simulink subsystem "Batteri"  (R2020b)
settings: Solver=VariableStepAuto  StartTime=0.0  StopTime=10.0  RelTol=1e-3
libraries: fl_lib x76, ee_lib x27, nesl_utility x2
(part 1 of 2)
settings Model: Creator=David  LastModifiedBy=Sixten

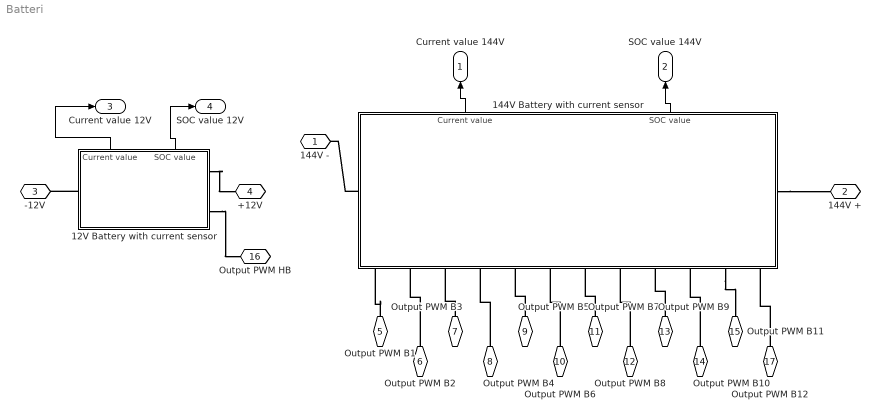
== system Batteri ==
  " 144V Battery with current sensor" : Subsystem
      settings: PortSchema="{\"entries\":[{\"content\":{\"sides\":[{\"content\":{\"connectorIds\":[\"LConn1\"]},\"type\":\"ConnectorPlacement.EquallySpacedRectSide\",\"uuid\":\"de94b407-ac45-4158-bf87-f7f71205b953\"},{\"content\":{\"connectorIds\":[\"RConn1\"],\"side\":\"RIGHT\"},\"type\":\"ConnectorPlacement.EquallySpacedRectSide\",\"uuid\":\"5f37bfd3-1f83-41a2-8e4c-c028e2b46b1f\"},{\"content\":{\"connectorIds\":[\"Out1\",\"Out2\"],\"side\":\"TOP\"},\"type\":\"ConnectorPlacement.EquallySpacedRectSide\",\"uuid\":\"a2342012-b85c-4526-9142-351f25c37e79\"},{\"content\":{\"connectorIds\":[\"RConn2\",\"RConn3\",\"RConn4\",\"RConn5\",\"RConn6\",\"RConn7\",\"RConn8\",\"RConn9\",\"RConn10\",\"RConn11\",\"RConn12\",\"RConn13\"],\"side\":\"BOTTOM\"},\"type\":\"ConnectorPlacement.EquallySpacedRectSide\",\"uuid\":\"61a274a5-577d-4bb8-8dc8-b17a7a1decde\"},{\"content\":{\"connectorIds\":[],\"side\":\"HIDDEN\"},\"type\":\"ConnectorPlacement.EquallySpacedRectSide\",\"uuid\":\"c9b59ba9-0057-4e9f-a00a-12995deaa940\"}]},\"type\":\"ConnectorPlacement.EquallySpacedConnector\",\"uuid\":\"0aadbf9b-8ffe-4e11-88ee-655997b921c3\"}],\"packageUris\":[\"http://schema.mathworks.com/mf0/Connector/R2020b\"],\"version\":\"1.0\"}"
  12V Battery with current sensor : Subsystem
      settings: PortSchema="{\"entries\":[{\"content\":{\"sides\":[{\"content\":{\"connectorIds\":[\"LConn1\"]},\"type\":\"ConnectorPlacement.EquallySpacedRectSide\",\"uuid\":\"de94b407-ac45-4158-bf87-f7f71205b953\"},{\"content\":{\"connectorIds\":[\"RConn1\",\"RConn2\"],\"side\":\"RIGHT\"},\"type\":\"ConnectorPlacement.EquallySpacedRectSide\",\"uuid\":\"5f37bfd3-1f83-41a2-8e4c-c028e2b46b1f\"},{\"content\":{\"connectorIds\":[\"Out1\",\"Out2\"],\"side\":\"TOP\"},\"type\":\"ConnectorPlacement.EquallySpacedRectSide\",\"uuid\":\"a2342012-b85c-4526-9142-351f25c37e79\"},{\"content\":{\"connectorIds\":[],\"side\":\"BOTTOM\"},\"type\":\"ConnectorPlacement.EquallySpacedRectSide\",\"uuid\":\"fa1d5bca-3a30-4491-90b2-05abb2f1cee1\"},{\"content\":{\"connectorIds\":[],\"side\":\"HIDDEN\"},\"type\":\"ConnectorPlacement.EquallySpacedRectSide\",\"uuid\":\"c9b59ba9-0057-4e9f-a00a-12995deaa940\"}]},\"type\":\"ConnectorPlacement.EquallySpacedConnector\",\"uuid\":\"0aadbf9b-8ffe-4e11-88ee-655997b921c3\"}],\"packageUris\":[\"http://schema.mathworks.com/mf0/Connector/R2020b\"],\"version\":\"1.0\"}"
  144V - : PMIOPort  Side=Left
  144V + : PMIOPort  Port=2  Side=Right
  -12V : PMIOPort  Port=3  Side=Left
  +12V : PMIOPort  Port=4  Side=Right
  Output PWM B1 : PMIOPort  Port=5  Side=Right
  Output PWM B2 : PMIOPort  Port=6  Side=Right
  Output PWM B3 : PMIOPort  Port=7  Side=Right
  Output PWM B4 : PMIOPort  Port=8  Side=Right
  Output PWM B5 : PMIOPort  Port=9  Side=Right
  Output PWM B6 : PMIOPort  Port=10  Side=Right
  Output PWM B7 : PMIOPort  Port=11  Side=Right
  Output PWM B8 : PMIOPort  Port=12  Side=Right
  Output PWM B9 : PMIOPort  Port=13  Side=Right
  Output PWM B10 : PMIOPort  Port=14  Side=Right
  Output PWM B11 : PMIOPort  Port=15  Side=Right
  Output PWM HB : PMIOPort  Port=16  Side=Right
  Output PWM B12 : PMIOPort  Port=17  Side=Right
  Current value 144V : Outport
  SOC value 144V : Outport  Port=2
  Current value 12V : Outport  Port=3
  SOC value 12V : Outport  Port=4
  wires:
  " 144V Battery with current sensor"/1(Current value) -> Current value 144V/1
  12V Battery with current sensor/1(Current value) -> Current value 12V/1
  12V Battery with current sensor/2(SOC value) -> SOC value 12V/1
  " 144V Battery with current sensor"/2(SOC value) -> SOC value 144V/1
  connections:
  " 144V Battery with current sensor"/RConn1 -- 144V +/RConn1
  " 144V Battery with current sensor"/LConn1 -- 144V -/RConn1
  12V Battery with current sensor/LConn1 -- -12V/RConn1
  12V Battery with current sensor/RConn1 -- +12V/RConn1
  Output PWM B1/RConn1 -- " 144V Battery with current sensor"/RConn2
  Output PWM B2/RConn1 -- " 144V Battery with current sensor"/RConn3
  Output PWM B3/RConn1 -- " 144V Battery with current sensor"/RConn4
  Output PWM B4/RConn1 -- " 144V Battery with current sensor"/RConn5
  Output PWM B5/RConn1 -- " 144V Battery with current sensor"/RConn6
  Output PWM B6/RConn1 -- " 144V Battery with current sensor"/RConn7
  Output PWM B7/RConn1 -- " 144V Battery with current sensor"/RConn8
  Output PWM B8/RConn1 -- " 144V Battery with current sensor"/RConn9
  Output PWM B9/RConn1 -- " 144V Battery with current sensor"/RConn10
  Output PWM B10/RConn1 -- " 144V Battery with current sensor"/RConn11
  " 144V Battery with current sensor"/RConn12 -- Output PWM B11/RConn1
  12V Battery with current sensor/RConn2 -- Output PWM HB/RConn1
  Output PWM B12/RConn1 -- " 144V Battery with current sensor"/RConn13

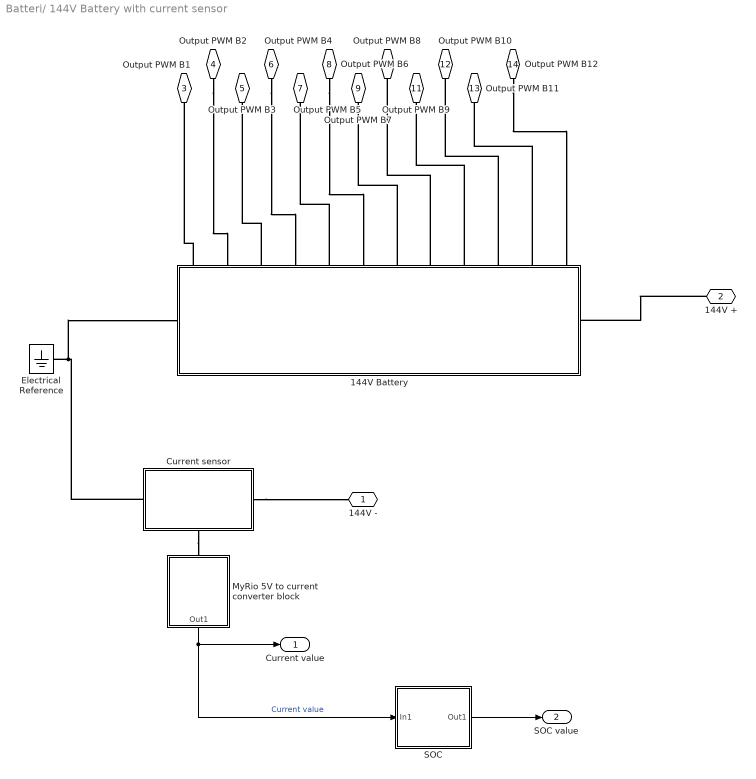
== system Batteri/ 144V Battery with current sensor ==
  " SOC" : Subsystem
  144V Battery : Subsystem
      settings: PortSchema="{\"entries\":[{\"content\":{\"sides\":[{\"content\":{\"connectorIds\":[\"LConn1\"]},\"type\":\"ConnectorPlacement.EquallySpacedRectSide\",\"uuid\":\"e99ced6f-69e8-4252-8471-6cdb96ceb2b2\"},{\"content\":{\"connectorIds\":[\"RConn1\"],\"side\":\"RIGHT\"},\"type\":\"ConnectorPlacement.EquallySpacedRectSide\",\"uuid\":\"43ce9788-4860-4398-aee6-6e594bef3b24\"},{\"content\":{\"connectorIds\":[\"LConn2\",\"LConn3\",\"LConn4\",\"LConn5\",\"LConn6\",\"LConn7\",\"LConn8\",\"LConn9\",\"LConn10\",\"LConn11\",\"LConn12\",\"LConn13\"],\"side\":\"TOP\"},\"type\":\"ConnectorPlacement.EquallySpacedRectSide\",\"uuid\":\"c38ed088-7784-4d04-84fd-2543a273ac23\"},{\"content\":{\"connectorIds\":[],\"side\":\"HIDDEN\"},\"type\":\"ConnectorPlacement.EquallySpacedRectSide\",\"uuid\":\"e037fcb5-e400-4ff2-9ee1-c6dab5a4f657\"}]},\"type\":\"ConnectorPlacement.EquallySpacedConnector\",\"uuid\":\"0126c910-ab8b-459c-9426-4e860af266e9\"}],\"packageUris\":[\"http://schema.mathworks.com/mf0/Connector/R2020b\"],\"version\":\"1.0\"}"
  Current sensor : Subsystem
      settings: PortSchema="{\"entries\":[{\"content\":{\"sides\":[{\"content\":{\"connectorIds\":[\"LConn1\"]},\"type\":\"ConnectorPlacement.EquallySpacedRectSide\",\"uuid\":\"83570808-fc29-4e6a-be28-aa8d0eabb79f\"},{\"content\":{\"connectorIds\":[\"RConn1\"],\"side\":\"RIGHT\"},\"type\":\"ConnectorPlacement.EquallySpacedRectSide\",\"uuid\":\"416c4cd8-a069-48b3-a3c7-74116419a4db\"},{\"content\":{\"connectorIds\":[],\"side\":\"TOP\"},\"type\":\"ConnectorPlacement.EquallySpacedRectSide\",\"uuid\":\"a4fb3738-5515-4a74-8adf-a2dd979befdd\"},{\"content\":{\"connectorIds\":[\"RConn2\"],\"side\":\"BOTTOM\"},\"type\":\"ConnectorPlacement.EquallySpacedRectSide\",\"uuid\":\"ad628acf-3503-4419-88b3-b3eb14bb30ce\"},{\"content\":{\"connectorIds\":[],\"side\":\"HIDDEN\"},\"type\":\"ConnectorPlacement.EquallySpacedRectSide\",\"uuid\":\"b744c287-8e60-4db7-938e-bc5b63a55d48\"}]},\"type\":\"ConnectorPlacement.EquallySpacedConnector\",\"uuid\":\"a4a86a7b-faa9-4dcc-948f-f4075230c4ff\"}],\"packageUris\":[\"http://schema.mathworks.com/mf0/Connector/R2020b\"],\"version\":\"1.0\"}"
  Electrical Reference : fl_lib/Electrical/Electrical Elements/Electrical Reference
  MyRio 5V to current converter block : Subsystem
  144V - : PMIOPort  Side=Left
  144V + : PMIOPort  Port=2  Side=Right
  Output PWM B1 : PMIOPort  Port=3  Side=Right
  Output PWM B2 : PMIOPort  Port=4  Side=Right
  Output PWM B3 : PMIOPort  Port=5  Side=Right
  Output PWM B4 : PMIOPort  Port=6  Side=Right
  Output PWM B5 : PMIOPort  Port=7  Side=Right
  Output PWM B6 : PMIOPort  Port=8  Side=Right
  Output PWM B7 : PMIOPort  Port=9  Side=Right
  Output PWM B8 : PMIOPort  Port=10  Side=Right
  Output PWM B9 : PMIOPort  Port=11  Side=Right
  Output PWM B10 : PMIOPort  Port=12  Side=Right
  Output PWM B11 : PMIOPort  Port=13  Side=Right
  Output PWM B12 : PMIOPort  Port=14  Side=Right
  Current value : Outport
  SOC value : Outport  Port=2
  wires:
  " SOC"/1(Out1) -> SOC value/1
  MyRio 5V to current converter block/1(Out1) -> Current value/1, " SOC"/1(In1)  "Current value"
  connections:
  Output PWM B12/RConn1 -- 144V Battery/LConn13
  Current sensor/RConn2 -- MyRio 5V to current converter block/LConn1
  144V +/RConn1 -- 144V Battery/RConn1
  Electrical Reference/LConn1 -- 144V Battery/LConn1 -- Current sensor/LConn1
  Current sensor/RConn1 -- 144V -/RConn1
  144V Battery/LConn2 -- Output PWM B1/RConn1
  Output PWM B2/RConn1 -- 144V Battery/LConn3
  144V Battery/LConn4 -- Output PWM B3/RConn1
  Output PWM B4/RConn1 -- 144V Battery/LConn5
  144V Battery/LConn6 -- Output PWM B5/RConn1
  Output PWM B6/RConn1 -- 144V Battery/LConn7
  144V Battery/LConn8 -- Output PWM B7/RConn1
  144V Battery/LConn9 -- Output PWM B8/RConn1
  144V Battery/LConn10 -- Output PWM B9/RConn1
  144V Battery/LConn11 -- Output PWM B10/RConn1
  144V Battery/LConn12 -- Output PWM B11/RConn1

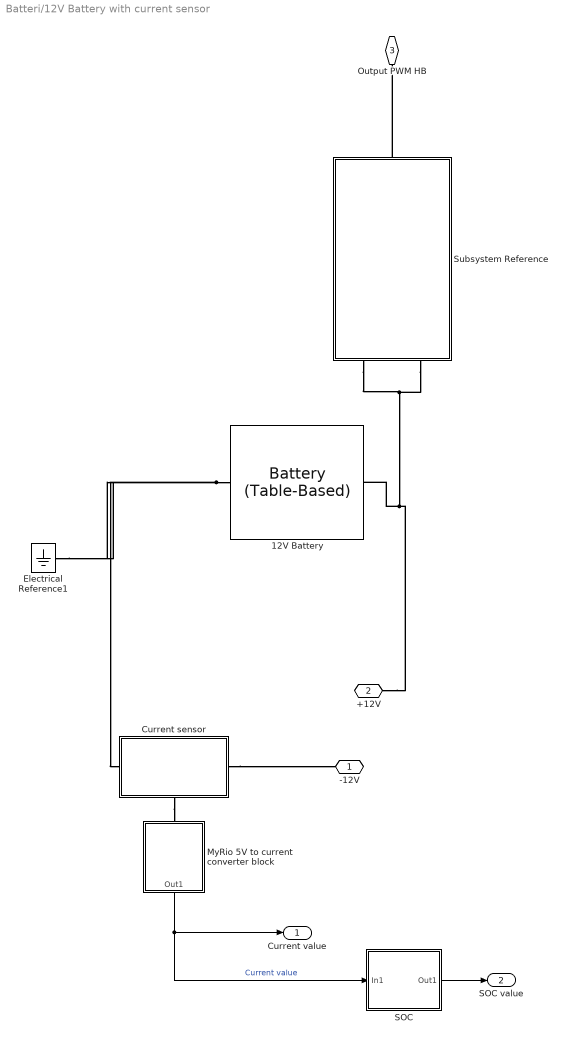
== system Batteri/12V Battery with current sensor ==
  " SOC" : Subsystem
  12V Battery : ee_lib/Sources/Battery (Table-Based)  SOC_vec=[0, .25, 0.5, .75, 1]  T_dependence=ee.enum.temperature_dependence.no  prm_dir=ee.enum.battery.prm_dir.noCurrentDirectionality  T_vec=[273.15, 298.15, 323.15] K  V0_mat=[3.2, 3.1, 3.14; 3.25, 3.27, 3.3; 3.28, 3.31, 3.34; 3.33, 3.5, 3.59] V  V0_vec=[11.7, 12, 12.2, 12.4, 12.8] V  R0_mat=[.03, .015, .002; .04, .017, .008; .039, .012, .006; .027, .013, .021] Ohm  R0_vec=[0.0055, 0.0055, 0.0055, 0.0055, 0.0055] Ohm  R0_dis_mat=[.03, .015, .002; .04, .017, .008; .039, .012, .006; .027, .013, .021] Ohm  R0_dis_vec=[.015, .017, .012, .013] Ohm  R0_ch_mat=[.03, .015, .002; .04, .017, .008; .039, .012, .006; .027, .013, .021] Ohm  R0_ch_vec=[.015, .017, .012, .013] Ohm  AH_vec=[2.9, 4.1, 4.2] hr*A  AH=70 hr*A  prm_leak=ee.enum.battery.prm_leak.disabled  Rleak_vec=[8000, 7000, 6000] Ohm  Rleak=7e3 Ohm  extrapolation_option=ee.enum.extrapolation.linear  prm_dyn=ee.enum.battery.prm_dyn.off  R1_mat=[.089, .076, .01; .042, .022, .099; .019, .007, .002; .051, .043, .029] Ohm  R1_vec=[.076, .022, .007, .043] Ohm  tau1_mat=[44, 148, 235; 93, 110, 1000; 19, 27, 133; .5, 22, 3] s  tau1_vec=[148, 110, 27, 22] s  R2_mat=[.014, .382, .407; .028, .006, .007; .014, .007, .006; .333, .956, .912] Ohm  R2_vec=[.382, .006, .007, .956] Ohm  tau2_mat=[1, 44, 5644; 11, 24, 506; 2, 14, 330; 3310, 13419, 30216] s  tau2_vec=[44, 24, 14, 13419] s  R3_mat=[.014, .382, .407; .028, .006, .007; .014, .007, .006; .333, .956, .912] Ohm  R3_vec=[.382, .006, .007, .956] Ohm  tau3_mat=[1, 44, 5644; 11, 24, 506; 2, 14, 330; 3310, 13419, 30216] s  tau3_vec=[44, 24, 14, 13419] s  R4_mat=[.014, .382, .407; .028, .006, .007; .014, .007, .006; .333, .956, .912] Ohm  R4_vec=[.382, .006, .007, .956] Ohm  tau4_mat=[1, 44, 5644; 11, 24, 506; 2, 14, 330; 3310, 13419, 30216] s  tau4_vec=[44, 24, 14, 13419] s  R5_mat=[.014, .382, .407; .028, .006, .007; .014, .007, .006; .333, .956, .912] Ohm  R5_vec=[.382, .006, .007, .956] Ohm  tau5_mat=[1, 44, 5644; 11, 24, 506; 2, 14, 330; 3310, 13419, 30216] s  tau5_vec=[44, 24, 14, 13419] s  prm_fade=ee.enum.battery.prm_fade.equations  N0=100  dV0=0  dR0=0  dAH=0  dRleak=0  dR1=0  dR2=0  dR3=0  dR4=0  dR5=0  N0vec=[100, 200, 300]  Tfadevec=[298.15, 323.15] K  dV0vec=[0, 0, 0]  dR0vec=[0, 0, 0]  dAHvec=[0, 0, 0]  dRleakvec=[0, 0, 0]  dR1vec=[0, 0, 0]  dR2vec=[0, 0, 0]  dR3vec=[0, 0, 0]  dR4vec=[0, 0, 0]  dR5vec=[0, 0, 0]  dV0mat=[0, 0; 0, 0; 0, 0]  dR0mat=[0, 0; 0, 0; 0, 0]  dAHmat=[0, 0; 0, 0; 0, 0]  dRleakmat=[0, 0; 0, 0; 0, 0]  dR1mat=[0, 0; 0, 0; 0, 0]  dR2mat=[0, 0; 0, 0; 0, 0]  dR3mat=[0, 0; 0, 0; 0, 0]  dR4mat=[0, 0; 0, 0; 0, 0]  dR5mat=[0, 0; 0, 0; 0, 0]  temperature=298.15 K  i_specify=off  i_priority=None  i=0 A  i_nominal_specify=off  i_nominal_unit=A  i_nominal_value=1  v_specify=off  v_priority=None  v=0 V  v_nominal_specify=off  v_nominal_unit=V  v_nominal_value=1  stateOfCharge_specify=off  stateOfCharge_priority=High  stateOfCharge=1  stateOfCharge_nominal_specify=off  stateOfCharge_nominal_unit=1  stateOfCharge_nominal_value=1  num_cycles_specify=off  num_cycles_priority=High  num_cycles=0  num_cycles_nominal_specify=off  num_cycles_nominal_unit=1  num_cycles_nominal_value=1  thermal_mass=30000 J/K  temperature_specify=off  temperature_priority=High  temperature_nominal_specify=off  temperature_nominal_unit=K  temperature_nominal_value=1
      settings: SourceProductBaseCode=PS  InternalSimscapePortConfiguration="{\"Bottom\":[],\"Left\":[{\"id\":\"p\",\"label\":\"+\",\"type\":\"foundation.electrical.electrical\"}],\"Right\":[{\"id\":\"n\",\"label\":\"-\",\"type\":\"foundation.electrical.electrical\"}],\"Top\":[]}"
  Current sensor : Subsystem
      settings: PortSchema="{\"entries\":[{\"content\":{\"sides\":[{\"content\":{\"connectorIds\":[\"LConn1\"]},\"type\":\"ConnectorPlacement.EquallySpacedRectSide\",\"uuid\":\"83570808-fc29-4e6a-be28-aa8d0eabb79f\"},{\"content\":{\"connectorIds\":[\"RConn1\"],\"side\":\"RIGHT\"},\"type\":\"ConnectorPlacement.EquallySpacedRectSide\",\"uuid\":\"416c4cd8-a069-48b3-a3c7-74116419a4db\"},{\"content\":{\"connectorIds\":[],\"side\":\"TOP\"},\"type\":\"ConnectorPlacement.EquallySpacedRectSide\",\"uuid\":\"a4fb3738-5515-4a74-8adf-a2dd979befdd\"},{\"content\":{\"connectorIds\":[\"RConn2\"],\"side\":\"BOTTOM\"},\"type\":\"ConnectorPlacement.EquallySpacedRectSide\",\"uuid\":\"ad628acf-3503-4419-88b3-b3eb14bb30ce\"},{\"content\":{\"connectorIds\":[],\"side\":\"HIDDEN\"},\"type\":\"ConnectorPlacement.EquallySpacedRectSide\",\"uuid\":\"b744c287-8e60-4db7-938e-bc5b63a55d48\"}]},\"type\":\"ConnectorPlacement.EquallySpacedConnector\",\"uuid\":\"a4a86a7b-faa9-4dcc-948f-f4075230c4ff\"}],\"packageUris\":[\"http://schema.mathworks.com/mf0/Connector/R2020b\"],\"version\":\"1.0\"}"
  Electrical Reference1 : fl_lib/Electrical/Electrical Elements/Electrical Reference
  MyRio 5V to current converter block : Subsystem
  Subsystem Reference : Subsystem  ReferencedSubsystem=PWM
  -12V : PMIOPort  Side=Left
  +12V : PMIOPort  Port=2  Side=Right
  Output PWM HB : PMIOPort  Port=3  Side=Right
  Current value : Outport
  SOC value : Outport  Port=2
  wires:
  " SOC"/1(Out1) -> SOC value/1
  MyRio 5V to current converter block/1(Out1) -> " SOC"/1(In1), Current value/1  "Current value"
  connections:
  Subsystem Reference/RConn1 -- Output PWM HB/RConn1
  12V Battery/RConn1 -- Current sensor/LConn1 -- Electrical Reference1/LConn1
  Current sensor/RConn1 -- -12V/RConn1
  Subsystem Reference/LConn2 -- Subsystem Reference/LConn1 -- +12V/RConn1 -- 12V Battery/LConn1
  Current sensor/RConn2 -- MyRio 5V to current converter block/LConn1

== system Batteri/ 144V Battery with current sensor/ SOC ==
  In1 : Inport
  SOC1 : Subsystem
  Out1 : Outport
  wires:
  In1/1 -> SOC1/1(Input)
  SOC1/1(Output) -> Out1/1

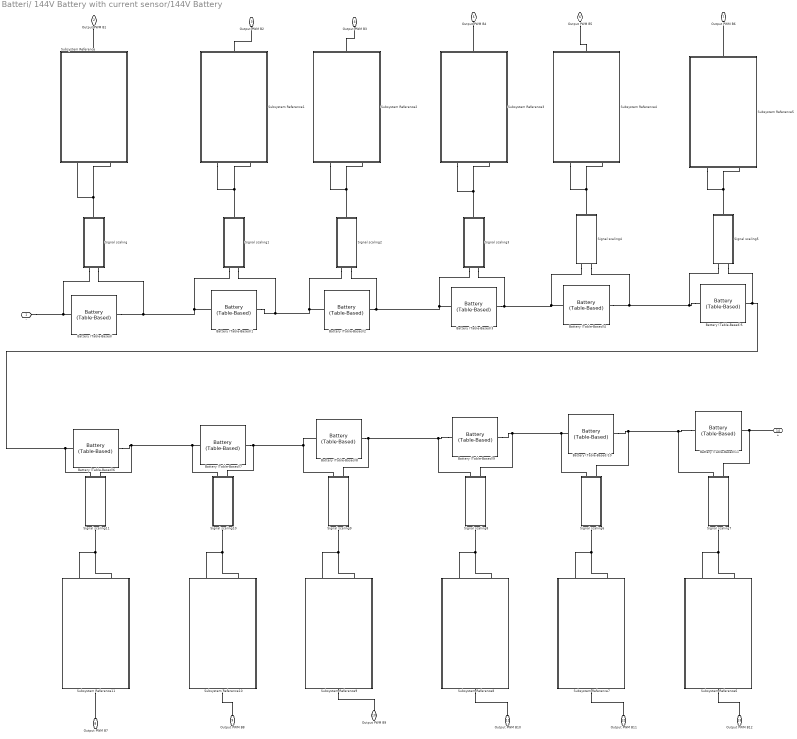
== system Batteri/ 144V Battery with current sensor/144V Battery ==
  Battery (Table-Based){,1..11} (12 alike) : ee_lib/Sources/Battery (Table-Based)  SOC_vec=[0, .25, 0.5, .75, 1]  T_dependence=ee.enum.temperature_dependence.no  prm_dir=ee.enum.battery.prm_dir.noCurrentDirectionality  T_vec=[273.15, 298.15, 323.15] K  V0_mat=[3.2, 3.1, 3.14; 3.25, 3.27, 3.3; 3.28, 3.31, 3.34; 3.33, 3.5, 3.59] V  V0_vec=[11.7, 12, 12.2, 12.4, 12.8] V  R0_mat=[.03, .015, .002; .04, .017, .008; .039, .012, .006; .027, .013, .021] Ohm  R0_vec=[0.0055, 0.0055, 0.0055, 0.0055, 0.0055] Ohm  R0_dis_mat=[.03, .015, .002; .04, .017, .008; .039, .012, .006; .027, .013, .021] Ohm  R0_dis_vec=[.015, .017, .012, .013] Ohm  R0_ch_mat=[.03, .015, .002; .04, .017, .008; .039, .012, .006; .027, .013, .021] Ohm  R0_ch_vec=[.015, .017, .012, .013] Ohm  AH_vec=[2.9, 4.1, 4.2] hr*A  AH=70 hr*A  prm_leak=ee.enum.battery.prm_leak.disabled  Rleak_vec=[8000, 7000, 6000] Ohm  Rleak=7e3 Ohm  extrapolation_option=ee.enum.extrapolation.linear  prm_dyn=ee.enum.battery.prm_dyn.off  R1_mat=[.089, .076, .01; .042, .022, .099; .019, .007, .002; .051, .043, .029] Ohm  R1_vec=[.076, .022, .007, .043] Ohm  tau1_mat=[44, 148, 235; 93, 110, 1000; 19, 27, 133; .5, 22, 3] s  tau1_vec=[148, 110, 27, 22] s  R2_mat=[.014, .382, .407; .028, .006, .007; .014, .007, .006; .333, .956, .912] Ohm  R2_vec=[.382, .006, .007, .956] Ohm  tau2_mat=[1, 44, 5644; 11, 24, 506; 2, 14, 330; 3310, 13419, 30216] s  tau2_vec=[44, 24, 14, 13419] s  R3_mat=[.014, .382, .407; .028, .006, .007; .014, .007, .006; .333, .956, .912] Ohm  R3_vec=[.382, .006, .007, .956] Ohm  tau3_mat=[1, 44, 5644; 11, 24, 506; 2, 14, 330; 3310, 13419, 30216] s  tau3_vec=[44, 24, 14, 13419] s  R4_mat=[.014, .382, .407; .028, .006, .007; .014, .007, .006; .333, .956, .912] Ohm  R4_vec=[.382, .006, .007, .956] Ohm  tau4_mat=[1, 44, 5644; 11, 24, 506; 2, 14, 330; 3310, 13419, 30216] s  tau4_vec=[44, 24, 14, 13419] s  R5_mat=[.014, .382, .407; .028, .006, .007; .014, .007, .006; .333, .956, .912] Ohm  R5_vec=[.382, .006, .007, .956] Ohm  tau5_mat=[1, 44, 5644; 11, 24, 506; 2, 14, 330; 3310, 13419, 30216] s  tau5_vec=[44, 24, 14, 13419] s  prm_fade=ee.enum.battery.prm_fade.equations  N0=100  dV0=0  dR0=0  dAH=0  dRleak=0  dR1=0  dR2=0  dR3=0  dR4=0  dR5=0  N0vec=[100, 200, 300]  Tfadevec=[298.15, 323.15] K  dV0vec=[0, 0, 0]  dR0vec=[0, 0, 0]  dAHvec=[0, 0, 0]  dRleakvec=[0, 0, 0]  dR1vec=[0, 0, 0]  dR2vec=[0, 0, 0]  dR3vec=[0, 0, 0]  dR4vec=[0, 0, 0]  dR5vec=[0, 0, 0]  dV0mat=[0, 0; 0, 0; 0, 0]  dR0mat=[0, 0; 0, 0; 0, 0]  dAHmat=[0, 0; 0, 0; 0, 0]  dRleakmat=[0, 0; 0, 0; 0, 0]  dR1mat=[0, 0; 0, 0; 0, 0]  dR2mat=[0, 0; 0, 0; 0, 0]  dR3mat=[0, 0; 0, 0; 0, 0]  dR4mat=[0, 0; 0, 0; 0, 0]  dR5mat=[0, 0; 0, 0; 0, 0]  temperature=298.15 K  i_specify=off  i_priority=None  i=0 A  i_nominal_specify=off  i_nominal_unit=A  i_nominal_value=1  v_specify=off  v_priority=None  v=0 V  v_nominal_specify=off  v_nominal_unit=V  v_nominal_value=1  stateOfCharge_specify=off  stateOfCharge_priority=High  stateOfCharge=1  stateOfCharge_nominal_specify=off  stateOfCharge_nominal_unit=1  stateOfCharge_nominal_value=1  num_cycles_specify=off  num_cycles_priority=High  num_cycles=0  num_cycles_nominal_specify=off  num_cycles_nominal_unit=1  num_cycles_nominal_value=1  thermal_mass=30000 J/K  temperature_specify=off  temperature_priority=High  temperature_nominal_specify=off  temperature_nominal_unit=K  temperature_nominal_value=1
      settings: SourceProductBaseCode=PS  InternalSimscapePortConfiguration="{\"Bottom\":[],\"Left\":[{\"id\":\"p\",\"label\":\"+\",\"type\":\"foundation.electrical.electrical\"}],\"Right\":[{\"id\":\"n\",\"label\":\"-\",\"type\":\"foundation.electrical.electrical\"}],\"Top\":[]}"
  Signal scaling : Subsystem
  Signal scaling1 : Subsystem
  Signal scaling10 : Subsystem
  Signal scaling11 : Subsystem
  Signal scaling2 : Subsystem
  Signal scaling3 : Subsystem
  Signal scaling4 : Subsystem
  Signal scaling5 : Subsystem
  Signal scaling6 : Subsystem
  Signal scaling7 : Subsystem
  Signal scaling8 : Subsystem
  Signal scaling9 : Subsystem
  Subsystem Reference{,1..11} (12 alike) : Subsystem  ReferencedSubsystem=PWM
  - : PMIOPort  Side=Left
  Output PWM B1 : PMIOPort  Port=2  Side=Left
  Output PWM B2 : PMIOPort  Port=3  Side=Left
  Output PWM B3 : PMIOPort  Port=4  Side=Left
  Output PWM B4 : PMIOPort  Port=5  Side=Left
  Output PWM B5 : PMIOPort  Port=6  Side=Left
  Output PWM B6 : PMIOPort  Port=7  Side=Left
  Output PWM B7 : PMIOPort  Port=8  Side=Left
  Output PWM B8 : PMIOPort  Port=9  Side=Left
  Output PWM B9 : PMIOPort  Port=10  Side=Left
  Output PWM B10 : PMIOPort  Port=11  Side=Left
  Output PWM B11 : PMIOPort  Port=12  Side=Left
  Output PWM B12 : PMIOPort  Port=13  Side=Left
  + : PMIOPort  Port=14  Side=Right
  connections:
  Subsystem Reference6/LConn2 -- Subsystem Reference6/LConn1 -- Signal scaling7/RConn1
  Subsystem Reference7/LConn2 -- Signal scaling6/RConn1 -- Subsystem Reference7/LConn1
  Subsystem Reference8/LConn2 -- Signal scaling8/RConn1 -- Subsystem Reference8/LConn1
  Subsystem Reference9/LConn2 -- Subsystem Reference9/LConn1 -- Signal scaling9/RConn1
  Subsystem Reference10/LConn2 -- Signal scaling10/RConn1 -- Subsystem Reference10/LConn1
  Subsystem Reference11/LConn2 -- Signal scaling11/RConn1 -- Subsystem Reference11/LConn1
  Subsystem Reference5/LConn1 -- Signal scaling5/RConn1 -- Subsystem Reference5/LConn2
  Subsystem Reference4/LConn1 -- Subsystem Reference4/LConn2 -- Signal scaling4/RConn1
  Subsystem Reference3/LConn1 -- Signal scaling3/RConn1 -- Subsystem Reference3/LConn2
  Subsystem Reference2/LConn1 -- Signal scaling2/RConn1 -- Subsystem Reference2/LConn2
  Subsystem Reference1/LConn2 -- Signal scaling1/RConn1 -- Subsystem Reference1/LConn1
  Signal scaling/RConn1 -- Subsystem Reference/LConn1 -- Subsystem Reference/LConn2
  Signal scaling10/LConn1 -- Battery (Table-Based)7/RConn1 -- Battery (Table-Based)6/LConn1 -- Signal scaling11/LConn2
  Signal scaling/LConn1 -- Battery (Table-Based)/RConn1 -- -/RConn1
  Battery (Table-Based)5/RConn1 -- Signal scaling5/LConn1 -- Battery (Table-Based)4/LConn1 -- Signal scaling4/LConn2
  Signal scaling4/LConn1 -- Battery (Table-Based)4/RConn1 -- Battery (Table-Based)3/LConn1 -- Signal scaling3/LConn2
  Signal scaling3/LConn1 -- Battery (Table-Based)3/RConn1 -- Battery (Table-Based)2/LConn1 -- Signal scaling2/LConn2
  Signal scaling6/LConn1 -- Battery (Table-Based)10/RConn1 -- Battery (Table-Based)9/LConn1 -- Signal scaling8/LConn2
  Battery (Table-Based)9/RConn1 -- Signal scaling8/LConn1 -- Battery (Table-Based)8/LConn1 -- Signal scaling9/LConn2
  Signal scaling7/LConn2 -- Battery (Table-Based)11/LConn1 -- +/RConn1
  Signal scaling2/LConn1 -- Battery (Table-Based)2/RConn1 -- Battery (Table-Based)1/LConn1 -- Signal scaling1/LConn2
  Signal scaling1/LConn1 -- Battery (Table-Based)1/RConn1 -- Battery (Table-Based)/LConn1 -- Signal scaling/LConn2
  Battery (Table-Based)11/RConn1 -- Signal scaling7/LConn1 -- Battery (Table-Based)10/LConn1 -- Signal scaling6/LConn2
  Signal scaling9/LConn1 -- Battery (Table-Based)8/RConn1 -- Battery (Table-Based)7/LConn1 -- Signal scaling10/LConn2
  Signal scaling11/LConn1 -- Battery (Table-Based)6/RConn1 -- Battery (Table-Based)5/LConn1 -- Signal scaling5/LConn2
  Output PWM B1/RConn1 -- Subsystem Reference/RConn1
  Subsystem Reference1/RConn1 -- Output PWM B2/RConn1
  Subsystem Reference2/RConn1 -- Output PWM B3/RConn1
  Output PWM B4/RConn1 -- Subsystem Reference3/RConn1
  Output PWM B5/RConn1 -- Subsystem Reference4/RConn1
  Subsystem Reference5/RConn1 -- Output PWM B6/RConn1
  Subsystem Reference11/RConn1 -- Output PWM B7/RConn1
  Subsystem Reference10/RConn1 -- Output PWM B8/RConn1
  Subsystem Reference9/RConn1 -- Output PWM B9/RConn1
  Subsystem Reference8/RConn1 -- Output PWM B10/RConn1
  Subsystem Reference7/RConn1 -- Output PWM B11/RConn1
  Subsystem Reference6/RConn1 -- Output PWM B12/RConn1

== system Batteri/ 144V Battery with current sensor/Current sensor ==
  Own current sensor : Subsystem
  Shunt_resistor : fl_lib/Electrical/Electrical Elements/Resistor  R=0.001 Ohm  i_specify=off  i_priority=None  i=0 A  i_nominal_specify=off  i_nominal_unit=A  i_nominal_value=1  v_specify=off  v_priority=None  v=0 V  v_nominal_specify=off  v_nominal_unit=V  v_nominal_value=1
  - : PMIOPort  Side=Left
  + : PMIOPort  Port=2  Side=Right
  5V output : PMIOPort  Port=3  Side=Right
  connections:
  Own current sensor/RConn1 -- 5V output/RConn1
  -/RConn1 -- Own current sensor/LConn1 -- Shunt_resistor/LConn1
  Shunt_resistor/RConn1 -- +/RConn1 -- Own current sensor/LConn2

== system Batteri/ 144V Battery with current sensor/MyRio 5V to current converter block ==
  MyRio constant : Gain  Gain=59.885
  PS-Simulink Converter4 : nesl_utility/PS-Simulink Converter  PhysicalDomain=network_engine_domain  SubClassName=ps_output  LeftPortType=input  RightPortType=output  PseudoPeriodic=off  Frequencies=[]  Unit=inherit  AffineConversion=off
  input : PMIOPort  Side=Left
  Out1 : Outport
  wires:
  PS-Simulink Converter4/1 -> MyRio constant/1
  MyRio constant/1 -> Out1/1
  connections:
  PS-Simulink Converter4/LConn1 -- input/RConn1

== system Batteri/12V Battery with current sensor/ SOC ==
  In1 : Inport
  SOC1 : Subsystem
  Out1 : Outport
  wires:
  In1/1 -> SOC1/1(Input)
  SOC1/1(Output) -> Out1/1

== system Batteri/12V Battery with current sensor/Current sensor ==
  Own current sensor : Subsystem
  Shunt_resistor : fl_lib/Electrical/Electrical Elements/Resistor  R=0.001 Ohm  i_specify=off  i_priority=None  i=0 A  i_nominal_specify=off  i_nominal_unit=A  i_nominal_value=1  v_specify=off  v_priority=None  v=0 V  v_nominal_specify=off  v_nominal_unit=V  v_nominal_value=1
  - : PMIOPort  Side=Left
  + : PMIOPort  Port=2  Side=Right
  5V output : PMIOPort  Port=3  Side=Right
  connections:
  Own current sensor/RConn1 -- 5V output/RConn1
  -/RConn1 -- Own current sensor/LConn1 -- Shunt_resistor/LConn1
  Shunt_resistor/RConn1 -- +/RConn1 -- Own current sensor/LConn2

== system Batteri/12V Battery with current sensor/MyRio 5V to current converter block ==
  MyRio constant : Gain  Gain=4.326
  PS-Simulink Converter4 : nesl_utility/PS-Simulink Converter  PhysicalDomain=network_engine_domain  SubClassName=ps_output  LeftPortType=input  RightPortType=output  PseudoPeriodic=off  Frequencies=[]  Unit=inherit  AffineConversion=off
  input : PMIOPort  Side=Left
  Out1 : Outport
  wires:
  PS-Simulink Converter4/1 -> MyRio constant/1
  MyRio constant/1 -> Out1/1
  connections:
  PS-Simulink Converter4/LConn1 -- input/RConn1

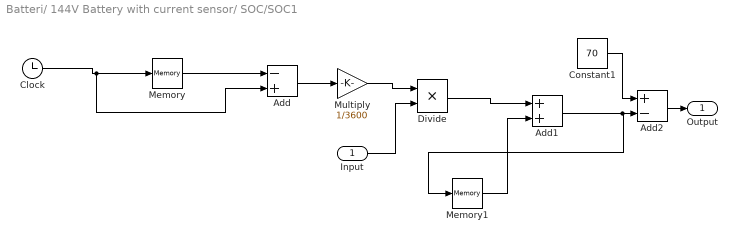
== system Batteri/ 144V Battery with current sensor/ SOC/SOC1 ==
  Input : Inport
  Add : Sum  Inputs=-+
  Add1 : Sum
  Add2 : Sum  Inputs=+-
  Clock : Clock
  Constant1 : Constant  Value=70  SampleTime=-1
  Divide : Product  Inputs=**
  Memory : Memory
  Memory1 : Memory
  Multiply : Gain  Gain=1/3600
  Output : Outport
  wires:
  Constant1/1 -> Add2/1
  Add2/1 -> Output/1
  Divide/1 -> Add1/1
  Multiply/1 -> Divide/1
  Input/1 -> Divide/2
  Add1/1 -> Add2/2, Memory1/1
  Memory1/1 -> Add1/2
  Add/1 -> Multiply/1
  Memory/1 -> Add/1
  Clock/1 -> Memory/1, Add/2

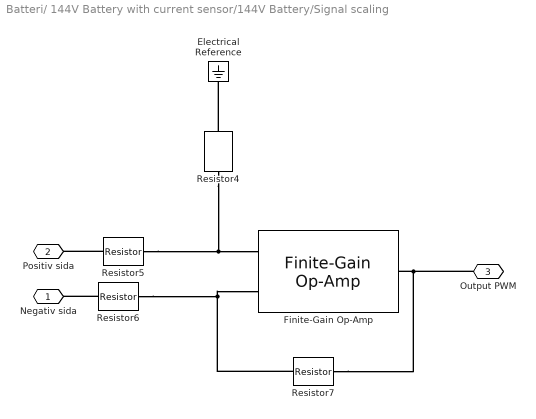
== system Batteri/ 144V Battery with current sensor/144V Battery/Signal scaling ==
  Electrical Reference : fl_lib/Electrical/Electrical Elements/Electrical Reference
  Finite-Gain Op-Amp : ee_lib/Integrated Circuits/Finite-Gain Op-Amp  A=1000  Rin=1e6 Ohm  Rout=0 Ohm  Vmin=-15 V  Vmax=15 V  noise_mode=0  v_noise=30e-9 V/Hz^0.50000  noise_prm=1  i_noise=0.5e-12 A/Hz^0.50000  ip_noise=0.5e-12 A/Hz^0.50000  in_noise=0.5e-12 A/Hz^0.50000  sample_time=1e-3 s  repeatability=1  auto_seed_v=1196140742  auto_seed_ip=2348838240  auto_seed_in=4112460543  user_seed_v=0  user_seed_ip=0  user_seed_in=0
      settings: SourceProductBaseCode=PS  InternalSimscapePortConfiguration="{\"Bottom\":[],\"Left\":[{\"id\":\"p\",\"label\":\"+\",\"type\":\"foundation.electrical.electrical\"},{\"id\":\"n\",\"label\":\"-\",\"type\":\"foundation.electrical.electrical\"}],\"Right\":[{\"id\":\"out\",\"label\":\"\",\"type\":\"foundation.electrical.electrical\"}],\"Top\":[]}"
  Resistor{4..7} (4 alike) : fl_lib/Electrical/Electrical Elements/Resistor  R=1000 Ohm  i_specify=off  i_priority=None  i=0 A  i_nominal_specify=off  i_nominal_unit=A  i_nominal_value=1  v_specify=off  v_priority=None  v=0 V  v_nominal_specify=off  v_nominal_unit=V  v_nominal_value=1
  Negativ sida : PMIOPort  Side=Left
  Positiv sida : PMIOPort  Port=2  Side=Left
  Output PWM : PMIOPort  Port=3  Side=Right
  connections:
  Resistor4/RConn1 -- Electrical Reference/LConn1
  Resistor5/LConn1 -- Positiv sida/RConn1
  Resistor6/LConn1 -- Negativ sida/RConn1
  Resistor7/RConn1 -- Output PWM/RConn1 -- Finite-Gain Op-Amp/RConn1
  Resistor6/RConn1 -- Resistor7/LConn1 -- Finite-Gain Op-Amp/LConn2
  Resistor4/LConn1 -- Finite-Gain Op-Amp/LConn1 -- Resistor5/RConn1

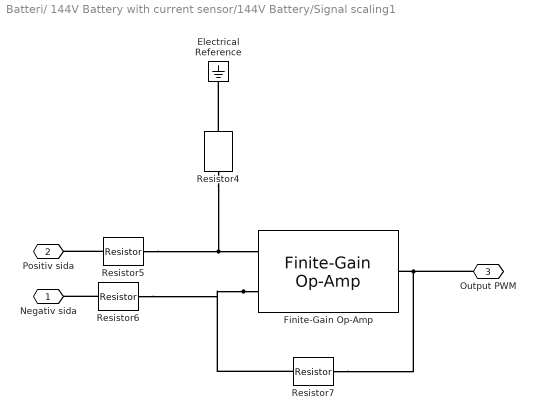
== system Batteri/ 144V Battery with current sensor/144V Battery/Signal scaling1 ==
  Electrical Reference : fl_lib/Electrical/Electrical Elements/Electrical Reference
  Finite-Gain Op-Amp : ee_lib/Integrated Circuits/Finite-Gain Op-Amp  A=1000  Rin=1e6 Ohm  Rout=0 Ohm  Vmin=-15 V  Vmax=15 V  noise_mode=0  v_noise=30e-9 V/Hz^0.50000  noise_prm=1  i_noise=0.5e-12 A/Hz^0.50000  ip_noise=0.5e-12 A/Hz^0.50000  in_noise=0.5e-12 A/Hz^0.50000  sample_time=1e-3 s  repeatability=1  auto_seed_v=4144164703  auto_seed_ip=676943032  auto_seed_in=4168664255  user_seed_v=0  user_seed_ip=0  user_seed_in=0
      settings: SourceProductBaseCode=PS  InternalSimscapePortConfiguration="{\"Bottom\":[],\"Left\":[{\"id\":\"p\",\"label\":\"+\",\"type\":\"foundation.electrical.electrical\"},{\"id\":\"n\",\"label\":\"-\",\"type\":\"foundation.electrical.electrical\"}],\"Right\":[{\"id\":\"out\",\"label\":\"\",\"type\":\"foundation.electrical.electrical\"}],\"Top\":[]}"
  Resistor{4..7} (4 alike) : fl_lib/Electrical/Electrical Elements/Resistor  R=1000 Ohm  i_specify=off  i_priority=None  i=0 A  i_nominal_specify=off  i_nominal_unit=A  i_nominal_value=1  v_specify=off  v_priority=None  v=0 V  v_nominal_specify=off  v_nominal_unit=V  v_nominal_value=1
  Negativ sida : PMIOPort  Side=Left
  Positiv sida : PMIOPort  Port=2  Side=Left
  Output PWM : PMIOPort  Port=3  Side=Right
  connections:
  Resistor5/RConn1 -- Finite-Gain Op-Amp/LConn1 -- Resistor4/LConn1
  Finite-Gain Op-Amp/LConn2 -- Resistor7/LConn1 -- Resistor6/RConn1
  Finite-Gain Op-Amp/RConn1 -- Output PWM/RConn1 -- Resistor7/RConn1
  Resistor6/LConn1 -- Negativ sida/RConn1
  Resistor5/LConn1 -- Positiv sida/RConn1
  Resistor4/RConn1 -- Electrical Reference/LConn1

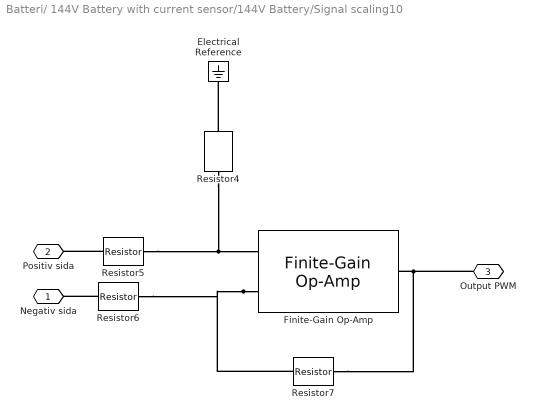
== system Batteri/ 144V Battery with current sensor/144V Battery/Signal scaling10 ==
  Electrical Reference : fl_lib/Electrical/Electrical Elements/Electrical Reference
  Finite-Gain Op-Amp : ee_lib/Integrated Circuits/Finite-Gain Op-Amp  A=1000  Rin=1e6 Ohm  Rout=0 Ohm  Vmin=-15 V  Vmax=15 V  noise_mode=0  v_noise=30e-9 V/Hz^0.50000  noise_prm=1  i_noise=0.5e-12 A/Hz^0.50000  ip_noise=0.5e-12 A/Hz^0.50000  in_noise=0.5e-12 A/Hz^0.50000  sample_time=1e-3 s  repeatability=1  auto_seed_v=4111000739  auto_seed_ip=2084672538  auto_seed_in=3437178441  user_seed_v=0  user_seed_ip=0  user_seed_in=0
      settings: SourceProductBaseCode=PS  InternalSimscapePortConfiguration="{\"Bottom\":[],\"Left\":[{\"id\":\"p\",\"label\":\"+\",\"type\":\"foundation.electrical.electrical\"},{\"id\":\"n\",\"label\":\"-\",\"type\":\"foundation.electrical.electrical\"}],\"Right\":[{\"id\":\"out\",\"label\":\"\",\"type\":\"foundation.electrical.electrical\"}],\"Top\":[]}"
  Resistor{4..7} (4 alike) : fl_lib/Electrical/Electrical Elements/Resistor  R=1000 Ohm  i_specify=off  i_priority=None  i=0 A  i_nominal_specify=off  i_nominal_unit=A  i_nominal_value=1  v_specify=off  v_priority=None  v=0 V  v_nominal_specify=off  v_nominal_unit=V  v_nominal_value=1
  Negativ sida : PMIOPort  Side=Left
  Positiv sida : PMIOPort  Port=2  Side=Left
  Output PWM : PMIOPort  Port=3  Side=Right
  connections:
  Resistor5/RConn1 -- Finite-Gain Op-Amp/LConn1 -- Resistor4/LConn1
  Finite-Gain Op-Amp/LConn2 -- Resistor7/LConn1 -- Resistor6/RConn1
  Finite-Gain Op-Amp/RConn1 -- Output PWM/RConn1 -- Resistor7/RConn1
  Resistor6/LConn1 -- Negativ sida/RConn1
  Resistor5/LConn1 -- Positiv sida/RConn1
  Resistor4/RConn1 -- Electrical Reference/LConn1

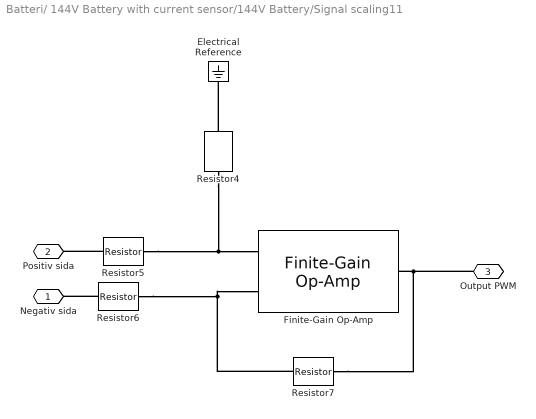
== system Batteri/ 144V Battery with current sensor/144V Battery/Signal scaling11 ==
  Electrical Reference : fl_lib/Electrical/Electrical Elements/Electrical Reference
  Finite-Gain Op-Amp : ee_lib/Integrated Circuits/Finite-Gain Op-Amp  A=1000  Rin=1e6 Ohm  Rout=0 Ohm  Vmin=-15 V  Vmax=15 V  noise_mode=0  v_noise=30e-9 V/Hz^0.50000  noise_prm=1  i_noise=0.5e-12 A/Hz^0.50000  ip_noise=0.5e-12 A/Hz^0.50000  in_noise=0.5e-12 A/Hz^0.50000  sample_time=1e-3 s  repeatability=1  auto_seed_v=609397185  auto_seed_ip=1811450916  auto_seed_in=3933054132  user_seed_v=0  user_seed_ip=0  user_seed_in=0
      settings: SourceProductBaseCode=PS  InternalSimscapePortConfiguration="{\"Bottom\":[],\"Left\":[{\"id\":\"p\",\"label\":\"+\",\"type\":\"foundation.electrical.electrical\"},{\"id\":\"n\",\"label\":\"-\",\"type\":\"foundation.electrical.electrical\"}],\"Right\":[{\"id\":\"out\",\"label\":\"\",\"type\":\"foundation.electrical.electrical\"}],\"Top\":[]}"
  Resistor{4..7} (4 alike) : fl_lib/Electrical/Electrical Elements/Resistor  R=1000 Ohm  i_specify=off  i_priority=None  i=0 A  i_nominal_specify=off  i_nominal_unit=A  i_nominal_value=1  v_specify=off  v_priority=None  v=0 V  v_nominal_specify=off  v_nominal_unit=V  v_nominal_value=1
  Negativ sida : PMIOPort  Side=Left
  Positiv sida : PMIOPort  Port=2  Side=Left
  Output PWM : PMIOPort  Port=3  Side=Right
  connections:
  Resistor4/RConn1 -- Electrical Reference/LConn1
  Resistor5/LConn1 -- Positiv sida/RConn1
  Resistor6/LConn1 -- Negativ sida/RConn1
  Resistor7/RConn1 -- Output PWM/RConn1 -- Finite-Gain Op-Amp/RConn1
  Resistor6/RConn1 -- Resistor7/LConn1 -- Finite-Gain Op-Amp/LConn2
  Resistor4/LConn1 -- Finite-Gain Op-Amp/LConn1 -- Resistor5/RConn1

== system Batteri/ 144V Battery with current sensor/144V Battery/Signal scaling2 ==
  Electrical Reference : fl_lib/Electrical/Electrical Elements/Electrical Reference
  Finite-Gain Op-Amp : ee_lib/Integrated Circuits/Finite-Gain Op-Amp  A=1000  Rin=1e6 Ohm  Rout=0 Ohm  Vmin=-15 V  Vmax=15 V  noise_mode=0  v_noise=30e-9 V/Hz^0.50000  noise_prm=1  i_noise=0.5e-12 A/Hz^0.50000  ip_noise=0.5e-12 A/Hz^0.50000  in_noise=0.5e-12 A/Hz^0.50000  sample_time=1e-3 s  repeatability=1  auto_seed_v=3402504572  auto_seed_ip=4120988592  auto_seed_in=2816384857  user_seed_v=0  user_seed_ip=0  user_seed_in=0
      settings: SourceProductBaseCode=PS  InternalSimscapePortConfiguration="{\"Bottom\":[],\"Left\":[{\"id\":\"p\",\"label\":\"+\",\"type\":\"foundation.electrical.electrical\"},{\"id\":\"n\",\"label\":\"-\",\"type\":\"foundation.electrical.electrical\"}],\"Right\":[{\"id\":\"out\",\"label\":\"\",\"type\":\"foundation.electrical.electrical\"}],\"Top\":[]}"
  Resistor{4..7} (4 alike) : fl_lib/Electrical/Electrical Elements/Resistor  R=1000 Ohm  i_specify=off  i_priority=None  i=0 A  i_nominal_specify=off  i_nominal_unit=A  i_nominal_value=1  v_specify=off  v_priority=None  v=0 V  v_nominal_specify=off  v_nominal_unit=V  v_nominal_value=1
  Negativ sida : PMIOPort  Side=Left
  Positiv sida : PMIOPort  Port=2  Side=Left
  Output PWM : PMIOPort  Port=3  Side=Right
  connections:
  Resistor4/RConn1 -- Electrical Reference/LConn1
  Resistor5/LConn1 -- Positiv sida/RConn1
  Resistor6/LConn1 -- Negativ sida/RConn1
  Resistor7/RConn1 -- Output PWM/RConn1 -- Finite-Gain Op-Amp/RConn1
  Resistor6/RConn1 -- Resistor7/LConn1 -- Finite-Gain Op-Amp/LConn2
  Resistor4/LConn1 -- Finite-Gain Op-Amp/LConn1 -- Resistor5/RConn1

== system Batteri/ 144V Battery with current sensor/144V Battery/Signal scaling3 ==
  Electrical Reference : fl_lib/Electrical/Electrical Elements/Electrical Reference
  Finite-Gain Op-Amp : ee_lib/Integrated Circuits/Finite-Gain Op-Amp  A=1000  Rin=1e6 Ohm  Rout=0 Ohm  Vmin=-15 V  Vmax=15 V  noise_mode=0  v_noise=30e-9 V/Hz^0.50000  noise_prm=1  i_noise=0.5e-12 A/Hz^0.50000  ip_noise=0.5e-12 A/Hz^0.50000  in_noise=0.5e-12 A/Hz^0.50000  sample_time=1e-3 s  repeatability=1  auto_seed_v=153380492  auto_seed_ip=3646982598  auto_seed_in=4011470453  user_seed_v=0  user_seed_ip=0  user_seed_in=0
      settings: SourceProductBaseCode=PS  InternalSimscapePortConfiguration="{\"Bottom\":[],\"Left\":[{\"id\":\"p\",\"label\":\"+\",\"type\":\"foundation.electrical.electrical\"},{\"id\":\"n\",\"label\":\"-\",\"type\":\"foundation.electrical.electrical\"}],\"Right\":[{\"id\":\"out\",\"label\":\"\",\"type\":\"foundation.electrical.electrical\"}],\"Top\":[]}"
  Resistor{4..7} (4 alike) : fl_lib/Electrical/Electrical Elements/Resistor  R=1000 Ohm  i_specify=off  i_priority=None  i=0 A  i_nominal_specify=off  i_nominal_unit=A  i_nominal_value=1  v_specify=off  v_priority=None  v=0 V  v_nominal_specify=off  v_nominal_unit=V  v_nominal_value=1
  Negativ sida : PMIOPort  Side=Left
  Positiv sida : PMIOPort  Port=2  Side=Left
  Output PWM : PMIOPort  Port=3  Side=Right
  connections:
  Resistor5/RConn1 -- Finite-Gain Op-Amp/LConn1 -- Resistor4/LConn1
  Finite-Gain Op-Amp/LConn2 -- Resistor7/LConn1 -- Resistor6/RConn1
  Finite-Gain Op-Amp/RConn1 -- Output PWM/RConn1 -- Resistor7/RConn1
  Resistor6/LConn1 -- Negativ sida/RConn1
  Resistor5/LConn1 -- Positiv sida/RConn1
  Resistor4/RConn1 -- Electrical Reference/LConn1

== system Batteri/ 144V Battery with current sensor/144V Battery/Signal scaling4 ==
  Electrical Reference : fl_lib/Electrical/Electrical Elements/Electrical Reference
  Finite-Gain Op-Amp : ee_lib/Integrated Circuits/Finite-Gain Op-Amp  A=1000  Rin=1e6 Ohm  Rout=0 Ohm  Vmin=-15 V  Vmax=15 V  noise_mode=0  v_noise=30e-9 V/Hz^0.50000  noise_prm=1  i_noise=0.5e-12 A/Hz^0.50000  ip_noise=0.5e-12 A/Hz^0.50000  in_noise=0.5e-12 A/Hz^0.50000  sample_time=1e-3 s  repeatability=1  auto_seed_v=2915145293  auto_seed_ip=3254469079  auto_seed_in=3191729647  user_seed_v=0  user_seed_ip=0  user_seed_in=0
      settings: SourceProductBaseCode=PS  InternalSimscapePortConfiguration="{\"Bottom\":[],\"Left\":[{\"id\":\"p\",\"label\":\"+\",\"type\":\"foundation.electrical.electrical\"},{\"id\":\"n\",\"label\":\"-\",\"type\":\"foundation.electrical.electrical\"}],\"Right\":[{\"id\":\"out\",\"label\":\"\",\"type\":\"foundation.electrical.electrical\"}],\"Top\":[]}"
  Resistor{4..7} (4 alike) : fl_lib/Electrical/Electrical Elements/Resistor  R=1000 Ohm  i_specify=off  i_priority=None  i=0 A  i_nominal_specify=off  i_nominal_unit=A  i_nominal_value=1  v_specify=off  v_priority=None  v=0 V  v_nominal_specify=off  v_nominal_unit=V  v_nominal_value=1
  Negativ sida : PMIOPort  Side=Left
  Positiv sida : PMIOPort  Port=2  Side=Left
  Output PWM : PMIOPort  Port=3  Side=Right
  connections:
  Resistor4/RConn1 -- Electrical Reference/LConn1
  Resistor5/LConn1 -- Positiv sida/RConn1
  Resistor6/LConn1 -- Negativ sida/RConn1
  Resistor7/RConn1 -- Output PWM/RConn1 -- Finite-Gain Op-Amp/RConn1
  Resistor6/RConn1 -- Resistor7/LConn1 -- Finite-Gain Op-Amp/LConn2
  Resistor4/LConn1 -- Finite-Gain Op-Amp/LConn1 -- Resistor5/RConn1

== system Batteri/ 144V Battery with current sensor/144V Battery/Signal scaling5 ==
  Electrical Reference : fl_lib/Electrical/Electrical Elements/Electrical Reference
  Finite-Gain Op-Amp : ee_lib/Integrated Circuits/Finite-Gain Op-Amp  A=1000  Rin=1e6 Ohm  Rout=0 Ohm  Vmin=-15 V  Vmax=15 V  noise_mode=0  v_noise=30e-9 V/Hz^0.50000  noise_prm=1  i_noise=0.5e-12 A/Hz^0.50000  ip_noise=0.5e-12 A/Hz^0.50000  in_noise=0.5e-12 A/Hz^0.50000  sample_time=1e-3 s  repeatability=1  auto_seed_v=1684602222  auto_seed_ip=2815256101  auto_seed_in=735241226  user_seed_v=0  user_seed_ip=0  user_seed_in=0
      settings: SourceProductBaseCode=PS  InternalSimscapePortConfiguration="{\"Bottom\":[],\"Left\":[{\"id\":\"p\",\"label\":\"+\",\"type\":\"foundation.electrical.electrical\"},{\"id\":\"n\",\"label\":\"-\",\"type\":\"foundation.electrical.electrical\"}],\"Right\":[{\"id\":\"out\",\"label\":\"\",\"type\":\"foundation.electrical.electrical\"}],\"Top\":[]}"
  Resistor{4..7} (4 alike) : fl_lib/Electrical/Electrical Elements/Resistor  R=1000 Ohm  i_specify=off  i_priority=None  i=0 A  i_nominal_specify=off  i_nominal_unit=A  i_nominal_value=1  v_specify=off  v_priority=None  v=0 V  v_nominal_specify=off  v_nominal_unit=V  v_nominal_value=1
  Negativ sida : PMIOPort  Side=Left
  Positiv sida : PMIOPort  Port=2  Side=Left
  Output PWM : PMIOPort  Port=3  Side=Right
  connections:
  Resistor5/RConn1 -- Finite-Gain Op-Amp/LConn1 -- Resistor4/LConn1
  Finite-Gain Op-Amp/LConn2 -- Resistor7/LConn1 -- Resistor6/RConn1
  Finite-Gain Op-Amp/RConn1 -- Output PWM/RConn1 -- Resistor7/RConn1
  Resistor6/LConn1 -- Negativ sida/RConn1
  Resistor5/LConn1 -- Positiv sida/RConn1
  Resistor4/RConn1 -- Electrical Reference/LConn1

== system Batteri/ 144V Battery with current sensor/144V Battery/Signal scaling6 ==
  Electrical Reference : fl_lib/Electrical/Electrical Elements/Electrical Reference
  Finite-Gain Op-Amp : ee_lib/Integrated Circuits/Finite-Gain Op-Amp  A=1000  Rin=1e6 Ohm  Rout=0 Ohm  Vmin=-15 V  Vmax=15 V  noise_mode=0  v_noise=30e-9 V/Hz^0.50000  noise_prm=1  i_noise=0.5e-12 A/Hz^0.50000  ip_noise=0.5e-12 A/Hz^0.50000  in_noise=0.5e-12 A/Hz^0.50000  sample_time=1e-3 s  repeatability=1  auto_seed_v=3032444857  auto_seed_ip=136721035  auto_seed_in=1189375164  user_seed_v=0  user_seed_ip=0  user_seed_in=0
      settings: SourceProductBaseCode=PS  InternalSimscapePortConfiguration="{\"Bottom\":[],\"Left\":[{\"id\":\"p\",\"label\":\"+\",\"type\":\"foundation.electrical.electrical\"},{\"id\":\"n\",\"label\":\"-\",\"type\":\"foundation.electrical.electrical\"}],\"Right\":[{\"id\":\"out\",\"label\":\"\",\"type\":\"foundation.electrical.electrical\"}],\"Top\":[]}"
  Resistor{4..7} (4 alike) : fl_lib/Electrical/Electrical Elements/Resistor  R=1000 Ohm  i_specify=off  i_priority=None  i=0 A  i_nominal_specify=off  i_nominal_unit=A  i_nominal_value=1  v_specify=off  v_priority=None  v=0 V  v_nominal_specify=off  v_nominal_unit=V  v_nominal_value=1
  Negativ sida : PMIOPort  Side=Left
  Positiv sida : PMIOPort  Port=2  Side=Left
  Output PWM : PMIOPort  Port=3  Side=Right
  connections:
  Resistor4/RConn1 -- Electrical Reference/LConn1
  Resistor5/LConn1 -- Positiv sida/RConn1
  Resistor6/LConn1 -- Negativ sida/RConn1
  Resistor7/RConn1 -- Output PWM/RConn1 -- Finite-Gain Op-Amp/RConn1
  Resistor6/RConn1 -- Resistor7/LConn1 -- Finite-Gain Op-Amp/LConn2
  Resistor4/LConn1 -- Finite-Gain Op-Amp/LConn1 -- Resistor5/RConn1

== system Batteri/ 144V Battery with current sensor/144V Battery/Signal scaling7 ==
  Electrical Reference : fl_lib/Electrical/Electrical Elements/Electrical Reference
  Finite-Gain Op-Amp : ee_lib/Integrated Circuits/Finite-Gain Op-Amp  A=1000  Rin=1e6 Ohm  Rout=0 Ohm  Vmin=-15 V  Vmax=15 V  noise_mode=0  v_noise=30e-9 V/Hz^0.50000  noise_prm=1  i_noise=0.5e-12 A/Hz^0.50000  ip_noise=0.5e-12 A/Hz^0.50000  in_noise=0.5e-12 A/Hz^0.50000  sample_time=1e-3 s  repeatability=1  auto_seed_v=198304613  auto_seed_ip=417177824  auto_seed_in=3536724442  user_seed_v=0  user_seed_ip=0  user_seed_in=0
      settings: SourceProductBaseCode=PS  InternalSimscapePortConfiguration="{\"Bottom\":[],\"Left\":[{\"id\":\"p\",\"label\":\"+\",\"type\":\"foundation.electrical.electrical\"},{\"id\":\"n\",\"label\":\"-\",\"type\":\"foundation.electrical.electrical\"}],\"Right\":[{\"id\":\"out\",\"label\":\"\",\"type\":\"foundation.electrical.electrical\"}],\"Top\":[]}"
  Resistor{4..7} (4 alike) : fl_lib/Electrical/Electrical Elements/Resistor  R=1000 Ohm  i_specify=off  i_priority=None  i=0 A  i_nominal_specify=off  i_nominal_unit=A  i_nominal_value=1  v_specify=off  v_priority=None  v=0 V  v_nominal_specify=off  v_nominal_unit=V  v_nominal_value=1
  Negativ sida : PMIOPort  Side=Left
  Positiv sida : PMIOPort  Port=2  Side=Left
  Output PWM : PMIOPort  Port=3  Side=Right
  connections:
  Resistor5/RConn1 -- Finite-Gain Op-Amp/LConn1 -- Resistor4/LConn1
  Finite-Gain Op-Amp/LConn2 -- Resistor7/LConn1 -- Resistor6/RConn1
  Finite-Gain Op-Amp/RConn1 -- Output PWM/RConn1 -- Resistor7/RConn1
  Resistor6/LConn1 -- Negativ sida/RConn1
  Resistor5/LConn1 -- Positiv sida/RConn1
  Resistor4/RConn1 -- Electrical Reference/LConn1

== system Batteri/ 144V Battery with current sensor/144V Battery/Signal scaling8 ==
  Electrical Reference : fl_lib/Electrical/Electrical Elements/Electrical Reference
  Finite-Gain Op-Amp : ee_lib/Integrated Circuits/Finite-Gain Op-Amp  A=1000  Rin=1e6 Ohm  Rout=0 Ohm  Vmin=-15 V  Vmax=15 V  noise_mode=0  v_noise=30e-9 V/Hz^0.50000  noise_prm=1  i_noise=0.5e-12 A/Hz^0.50000  ip_noise=0.5e-12 A/Hz^0.50000  in_noise=0.5e-12 A/Hz^0.50000  sample_time=1e-3 s  repeatability=1  auto_seed_v=2984266212  auto_seed_ip=1361931897  auto_seed_in=4081172623  user_seed_v=0  user_seed_ip=0  user_seed_in=0
      settings: SourceProductBaseCode=PS  InternalSimscapePortConfiguration="{\"Bottom\":[],\"Left\":[{\"id\":\"p\",\"label\":\"+\",\"type\":\"foundation.electrical.electrical\"},{\"id\":\"n\",\"label\":\"-\",\"type\":\"foundation.electrical.electrical\"}],\"Right\":[{\"id\":\"out\",\"label\":\"\",\"type\":\"foundation.electrical.electrical\"}],\"Top\":[]}"
  Resistor{4..7} (4 alike) : fl_lib/Electrical/Electrical Elements/Resistor  R=1000 Ohm  i_specify=off  i_priority=None  i=0 A  i_nominal_specify=off  i_nominal_unit=A  i_nominal_value=1  v_specify=off  v_priority=None  v=0 V  v_nominal_specify=off  v_nominal_unit=V  v_nominal_value=1
  Negativ sida : PMIOPort  Side=Left
  Positiv sida : PMIOPort  Port=2  Side=Left
  Output PWM : PMIOPort  Port=3  Side=Right
  connections:
  Resistor5/RConn1 -- Finite-Gain Op-Amp/LConn1 -- Resistor4/LConn1
  Finite-Gain Op-Amp/LConn2 -- Resistor7/LConn1 -- Resistor6/RConn1
  Finite-Gain Op-Amp/RConn1 -- Output PWM/RConn1 -- Resistor7/RConn1
  Resistor6/LConn1 -- Negativ sida/RConn1
  Resistor5/LConn1 -- Positiv sida/RConn1
  Resistor4/RConn1 -- Electrical Reference/LConn1

== system Batteri/ 144V Battery with current sensor/144V Battery/Signal scaling9 ==
  Electrical Reference : fl_lib/Electrical/Electrical Elements/Electrical Reference
  Finite-Gain Op-Amp : ee_lib/Integrated Circuits/Finite-Gain Op-Amp  A=1000  Rin=1e6 Ohm  Rout=0 Ohm  Vmin=-15 V  Vmax=15 V  noise_mode=0  v_noise=30e-9 V/Hz^0.50000  noise_prm=1  i_noise=0.5e-12 A/Hz^0.50000  ip_noise=0.5e-12 A/Hz^0.50000  in_noise=0.5e-12 A/Hz^0.50000  sample_time=1e-3 s  repeatability=1  auto_seed_v=147944790  auto_seed_ip=1884392676  auto_seed_in=1638781095  user_seed_v=0  user_seed_ip=0  user_seed_in=0
      settings: SourceProductBaseCode=PS  InternalSimscapePortConfiguration="{\"Bottom\":[],\"Left\":[{\"id\":\"p\",\"label\":\"+\",\"type\":\"foundation.electrical.electrical\"},{\"id\":\"n\",\"label\":\"-\",\"type\":\"foundation.electrical.electrical\"}],\"Right\":[{\"id\":\"out\",\"label\":\"\",\"type\":\"foundation.electrical.electrical\"}],\"Top\":[]}"
  Resistor{4..7} (4 alike) : fl_lib/Electrical/Electrical Elements/Resistor  R=1000 Ohm  i_specify=off  i_priority=None  i=0 A  i_nominal_specify=off  i_nominal_unit=A  i_nominal_value=1  v_specify=off  v_priority=None  v=0 V  v_nominal_specify=off  v_nominal_unit=V  v_nominal_value=1
  Negativ sida : PMIOPort  Side=Left
  Positiv sida : PMIOPort  Port=2  Side=Left
  Output PWM : PMIOPort  Port=3  Side=Right
  connections:
  Resistor4/RConn1 -- Electrical Reference/LConn1
  Resistor5/LConn1 -- Positiv sida/RConn1
  Resistor6/LConn1 -- Negativ sida/RConn1
  Resistor7/RConn1 -- Output PWM/RConn1 -- Finite-Gain Op-Amp/RConn1
  Resistor6/RConn1 -- Resistor7/LConn1 -- Finite-Gain Op-Amp/LConn2
  Resistor4/LConn1 -- Finite-Gain Op-Amp/LConn1 -- Resistor5/RConn1

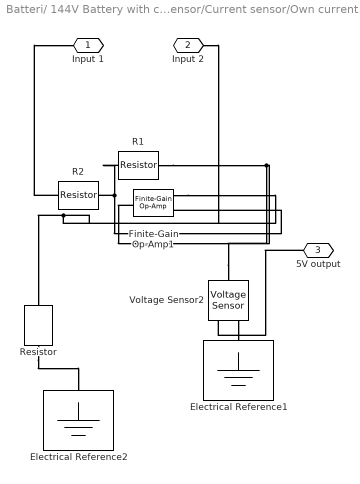
== system Batteri/ 144V Battery with current sensor/Current sensor/Own current sensor ==
  Electrical Reference1 : fl_lib/Electrical/Electrical Elements/Electrical Reference
  Electrical Reference2 : fl_lib/Electrical/Electrical Elements/Electrical Reference
  Finite-Gain Op-Amp1 : ee_lib/Integrated Circuits/Finite-Gain Op-Amp  A=1000  Rin=1e6 Ohm  Rout=0 Ohm  Vmin=0 V  Vmax=5 V  noise_mode=0  v_noise=30e-9 V/Hz^0.50000  noise_prm=1  i_noise=0.5e-12 A/Hz^0.50000  ip_noise=0.5e-12 A/Hz^0.50000  in_noise=0.5e-12 A/Hz^0.50000  sample_time=1e-3 s  repeatability=1  auto_seed_v=1582629291  auto_seed_ip=2687011258  auto_seed_in=3351051317  user_seed_v=0  user_seed_ip=0  user_seed_in=0
      settings: SourceProductBaseCode=PS  InternalSimscapePortConfiguration="{\"Bottom\":[],\"Left\":[{\"id\":\"p\",\"label\":\"+\",\"type\":\"foundation.electrical.electrical\"},{\"id\":\"n\",\"label\":\"-\",\"type\":\"foundation.electrical.electrical\"}],\"Right\":[{\"id\":\"out\",\"label\":\"\",\"type\":\"foundation.electrical.electrical\"}],\"Top\":[]}"
  R1 : fl_lib/Electrical/Electrical Elements/Resistor  R=16 Ohm  i_specify=off  i_priority=None  i=0 A  i_nominal_specify=off  i_nominal_unit=A  i_nominal_value=1  v_specify=off  v_priority=None  v=0 V  v_nominal_specify=off  v_nominal_unit=V  v_nominal_value=1
  R2 : fl_lib/Electrical/Electrical Elements/Resistor  R=1 Ohm  i_specify=off  i_priority=None  i=0 A  i_nominal_specify=off  i_nominal_unit=A  i_nominal_value=1  v_specify=off  v_priority=None  v=0 V  v_nominal_specify=off  v_nominal_unit=V  v_nominal_value=1
  Resistor : fl_lib/Electrical/Electrical Elements/Resistor  R=1 Ohm  i_specify=off  i_priority=None  i=0 A  i_nominal_specify=off  i_nominal_unit=A  i_nominal_value=1  v_specify=off  v_priority=None  v=0 V  v_nominal_specify=off  v_nominal_unit=V  v_nominal_value=1
  Voltage Sensor2 : fl_lib/Electrical/Electrical Sensors/Voltage Sensor
  Input 1 : PMIOPort  Side=Left
  Input 2 : PMIOPort  Port=2  Side=Left
  5V output : PMIOPort  Port=3  Side=Right
  connections:
  Resistor/RConn1 -- Electrical Reference2/LConn1
  R2/LConn1 -- Input 1/RConn1
  Voltage Sensor2/LConn1 -- Finite-Gain Op-Amp1/RConn1 -- R1/RConn1
  R1/LConn1 -- R2/RConn1 -- Finite-Gain Op-Amp1/LConn2
  Input 2/RConn1 -- Resistor/LConn1 -- Finite-Gain Op-Amp1/LConn1
  Voltage Sensor2/RConn2 -- Electrical Reference1/LConn1
  5V output/RConn1 -- Voltage Sensor2/RConn1

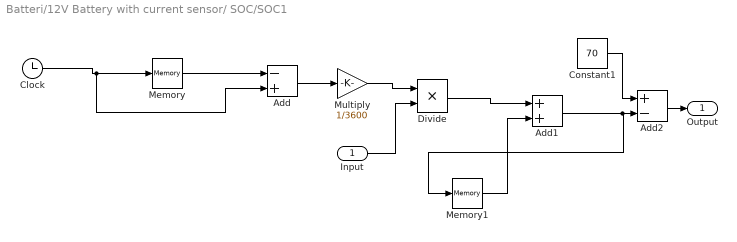
== system Batteri/12V Battery with current sensor/ SOC/SOC1 ==
  Input : Inport
  Add : Sum  Inputs=-+
  Add1 : Sum
  Add2 : Sum  Inputs=+-
  Clock : Clock
  Constant1 : Constant  Value=70  SampleTime=-1
  Divide : Product  Inputs=**
  Memory : Memory
  Memory1 : Memory
  Multiply : Gain  Gain=1/3600
  Output : Outport
  wires:
  Constant1/1 -> Add2/1
  Add2/1 -> Output/1
  Divide/1 -> Add1/1
  Multiply/1 -> Divide/1
  Input/1 -> Divide/2
  Add1/1 -> Add2/2, Memory1/1
  Memory1/1 -> Add1/2
  Add/1 -> Multiply/1
  Memory/1 -> Add/1
  Clock/1 -> Memory/1, Add/2
